simulink model "PID_Kim"  (R2016a)
settings: Solver=FixedStepAuto  StartTime=0.0  StopTime=10  FixedStep=0.01  RelTol=1e-3
values from neighbouring files (symbols this model uses):
  b = 10    [Tut_Week_4.m]    (also in Tut_week_2.m = [2;8;10])
  k = 20    [Tut_Week_4.m]    (also in Tut_week_7_Iden.m = 0.8)
  M = 1    [Tut_Week_4.m]    (also in Tut_week_4.m = [A ; -sin(th)  cos(th)])
settings Model: Creator=김태욱  LastModifiedBy=김태욱
settings DataIOCC: SaveFormat=Array  SaveState=on

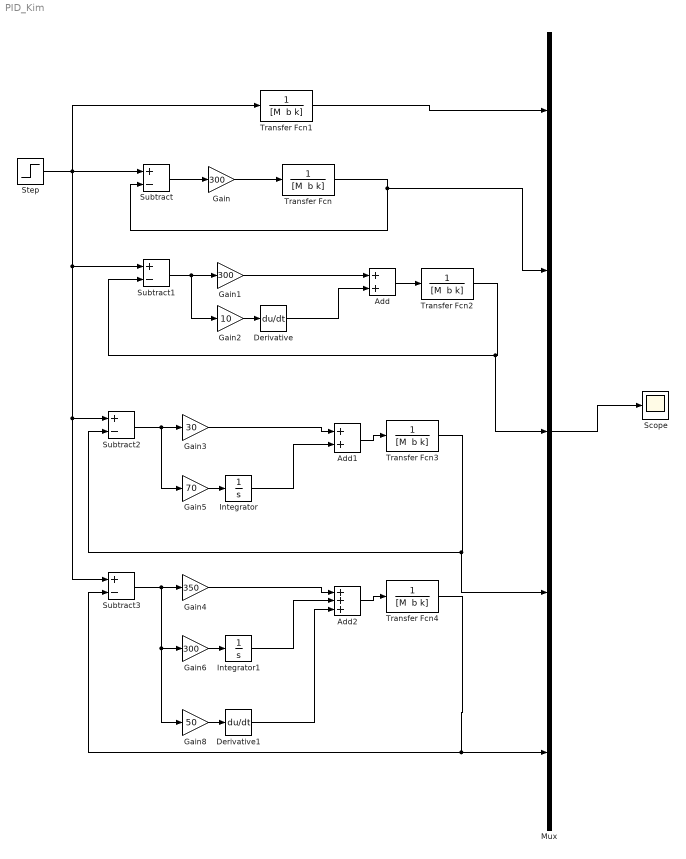
== system PID_Kim ==
  Add : Sum
  Add1 : Sum
  Add2 : Sum  Inputs=+++
  Derivative : Derivative
  Derivative1 : Derivative
  Gain : Gain  Gain=300
  Gain1 : Gain  Gain=300
  Gain2 : Gain  Gain=10
  Gain3 : Gain  Gain=30
  Gain4 : Gain  Gain=350
  Gain5 : Gain  Gain=70
  Gain6 : Gain  Gain=300
  Gain8 : Gain  Gain=50
  Integrator : Integrator
  Integrator1 : Integrator
  Mux : Mux  Inputs=5
  Scope : Scope
  Step : Step  SampleTime=0
  Subtract{,1..3} (4 alike) : Sum  Inputs=+-
  Transfer Fcn{,1..4} (5 alike) : TransferFcn  Denominator="[M  b k]"
  wires:
  Gain/1 -> Transfer Fcn/1
  Subtract/1 -> Gain/1
  Transfer Fcn/1 -> Mux/2, Subtract/2
  Transfer Fcn1/1 -> Mux/1
  Subtract1/1 -> Gain2/1, Gain1/1
  Gain2/1 -> Derivative/1
  Gain1/1 -> Add/1
  Derivative/1 -> Add/2
  Add/1 -> Transfer Fcn2/1
  Transfer Fcn2/1 -> Mux/3, Subtract1/2
  Subtract2/1 -> Gain5/1, Gain3/1
  Gain3/1 -> Add1/1
  Add1/1 -> Transfer Fcn3/1
  Transfer Fcn3/1 -> Mux/4, Subtract2/2
  Gain5/1 -> Integrator/1
  Integrator/1 -> Add1/2
  Mux/1 -> Scope/1
  Gain4/1 -> Add2/1
  Add2/1 -> Transfer Fcn4/1
  Transfer Fcn4/1 -> Subtract3/2, Mux/5
  Gain6/1 -> Integrator1/1
  Integrator1/1 -> Add2/2
  Step/1 -> Subtract1/1, Subtract3/1, Subtract2/1, Transfer Fcn1/1, Subtract/1
  Subtract3/1 -> Gain4/1, Gain8/1, Gain6/1
  Gain8/1 -> Derivative1/1
  Derivative1/1 -> Add2/3
